simulink model "simulink_both_machines_modified_moore"  (R2019b)
settings: Solver=VariableStepAuto  StartTime=0.0  StopTime=inf  RelTol=1e-3
settings Model: EnablePacing=on  PacingRate=0.250000  Creator=Bishoy Zaky  LastModifiedBy=Bishoy Zaky

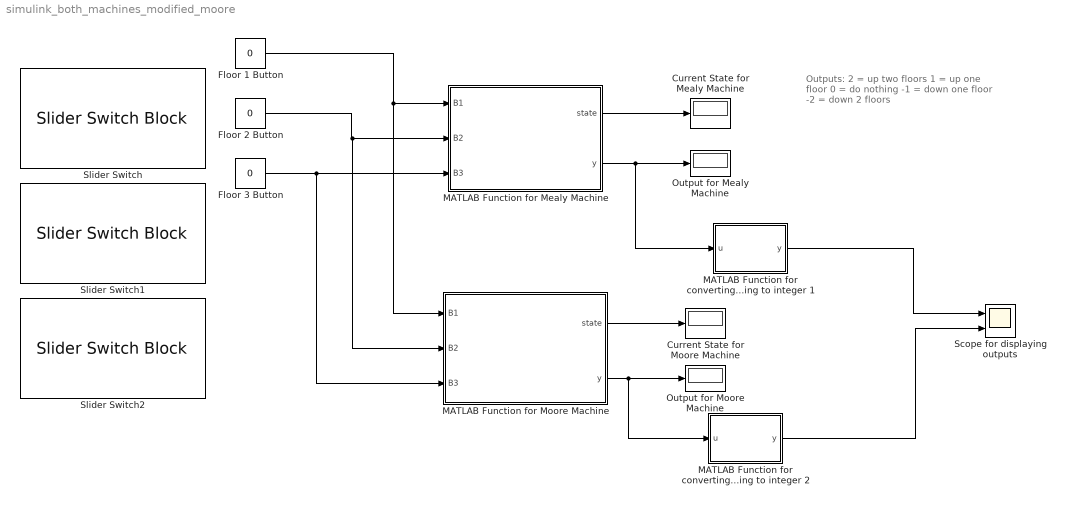
== system simulink_both_machines_modified_moore ==
  note: Outputs:
      | 2 = up two floors
      | 1 = up one floor
      | 0 = do nothing
      | -1 = down one floor
      | -2 = down 2 floors
  Current State for Mealy Machine : Display
  Current State for Moore Machine : Display
  Floor 1 Button : Constant  Value=0
  Floor 2 Button : Constant  Value=0
  Floor 3 Button : Constant  Value=0
  MATLAB Function for Mealy Machine : MATLAB Function  TreatAsAtomicUnit=on
  MATLAB Function for Moore Machine : MATLAB Function  TreatAsAtomicUnit=on
  MATLAB Function for converting output string to integer 1 : MATLAB Function  TreatAsAtomicUnit=on
  MATLAB Function for converting output string to integer 2 : MATLAB Function  TreatAsAtomicUnit=on
  Output for Mealy Machine : Display
  Output for Moore Machine : Display
  Scope for displaying outputs : Scope  NumInputPorts=2
  Slider Switch : SliderSwitchBlock
      settings: Values={{'Off', 'On'}, [0 1]}
  Slider Switch1 : SliderSwitchBlock
      settings: Values={{'Off', 'On'}, [0 1]}
  Slider Switch2 : SliderSwitchBlock
      settings: Values={{'Off', 'On'}, [0 1]}
  wires:
  Floor 1 Button/1 -> MATLAB Function for Moore Machine/1(B1), MATLAB Function for Mealy Machine/1(B1)
  MATLAB Function for converting output string to integer 1/1(y) -> Scope for displaying outputs/1
  Floor 2 Button/1 -> MATLAB Function for Moore Machine/2(B2), MATLAB Function for Mealy Machine/2(B2)
  MATLAB Function for Moore Machine/1(state) -> Current State for Moore Machine/1
  MATLAB Function for converting output string to integer 2/1(y) -> Scope for displaying outputs/2
  MATLAB Function for Mealy Machine/1(state) -> Current State for Mealy Machine/1
  Floor 3 Button/1 -> MATLAB Function for Moore Machine/3(B3), MATLAB Function for Mealy Machine/3(B3)
  MATLAB Function for Moore Machine/2(y) -> Output for Moore Machine/1, MATLAB Function for converting output string to integer 2/1(u)
  MATLAB Function for Mealy Machine/2(y) -> Output for Mealy Machine/1, MATLAB Function for converting output string to integer 1/1(u)

== matlab function simulink_both_machines_modified_moore/MATLAB Function for Moore Machine ==
  data: state output; B1 input; y output; B2 input; B3 input
function [state,y] = fcn(B1,B2,B3)
persistent current_state %state variable that persistes with every function call
if(isempty(current_state)) %initializing the state variable during first function call
    current_state = 1;
end
switch current_state 
    case 1 %state q1 represents being in the first floor
        if(B1) %B1, the first floor button, is pressed
            current_state = 1;
        elseif(B2) %B2, the second floor button, is pressed
            current_state = 4;
        elseif(B3) %B3, the third floor button, is pressed
            current_state = 6;
        end
    case 2 %state q2 represents being in the second floor
        if(B1)
            current_state = 5;
        elseif(B2)
            current_state = 2;
        elseif(B3)
            current_state = 4;
        end
    case 3 %state q3 represents being in the third floor
        if(B1) 
            current_state = 7;
        elseif(B2)
            current_state = 5;
        elseif(B3)
            current_state = 3;
        end
    case 4 %state q4 represents the transition state (first floor to second floor)
        if(B2)
            current_state = 2;
        elseif(B3)
            current_state = 3;
        elseif(B1)
            current_state = 4;
        end
    case 5 %state q5 represents the transition state (second floor to first floor)
        if(B1)
            current_state = 1;
        elseif(B2)
            current_state = 2;
        elseif(B3)
            current_state = 5;
        end
    case 6 %state q6 represents the transition state (first floor to third floor)
        if(B3)
            current_state = 3;
        elseif(B1)
            current_state = 6;    
        elseif(B2)
            current_state = 6;
        end  
    case 7 %state q7 represents the transition state (third floor to first floor)
        if(B1)
            current_state = 1;
        elseif(B2)
            current_state = 7;
        elseif(B3)
            current_state = 7;
        end
end
switch current_state %choose output depending on only the current state
    case 1 
        y = "s"; %elevator remains in place
    case 2
        y = "s";
    case 3
        y = "s";
    case 4
        y = "u1"; %elevator goes up 1 floor
    case 5
        y = "d1";
    case 6
        y = "u2"; %elevator goes up 2 floors
    otherwise
        y = "d2"; %elevator goes down 2 floors
end
state = current_state; %output current state
end

== matlab function simulink_both_machines_modified_moore/MATLAB Function for Mealy Machine ==
  data: state output; B1 input; y output; B2 input; B3 input
function [state,y] = fcn(B1,B2,B3)
persistent current_state %state variable that persistes with every function call
if(isempty(current_state)) %initializing the state variable during first function call
    current_state = 1;
end
switch current_state
    case 1  %state q1 represents being in the first floor
        if(B2) %B2, the second floor button, is pressed
            current_state = 2;
            y = "u1"; %elevator goes up 1 floor
        elseif(B3) %B3, the third floor button, is pressed
            current_state = 3;
            y = "u2"; %elevator goes up 2 floors
        else %B1, the first floor button, is pressed
            current_state = 1;
            y = "s"; %elevator remains in place
        end
    case 2  %state q2 represents being in the second floor
        if(B1)
            current_state = 1;
            y = "d1"; %elevator goes down 1 floor
        elseif(B3)
            current_state = 3;
            y = "u1"; %elevator goes up 1 floor
        else
            current_state = 2;
            y = "s"; %elevator remains in place
        end
    otherwise %otherwise state q3 represents being in the third floor
        if(B1)
            current_state = 1;
            y = "d2"; %elevator goes down 2 floors
        elseif(B2)
            current_state = 2;
            y = "d1"; %elevator goes down 1 floor
        else
            current_state = 3;
            y = "s"; %elevator remains in place
        end
end
state = current_state; %output current state
end

== matlab function simulink_both_machines_modified_moore/MATLAB Function for converting output string to integer 1 ==
  data: u input; y output
function y = fcn(u)
if u == "s"
    y = 0;
elseif u == "u1"
    y = 1;
elseif u == "u2"
    y = 2;
elseif u == "d1"
    y = -1;
else
    y = -2;
end

== matlab function simulink_both_machines_modified_moore/MATLAB Function for converting output string to integer 2 ==
  data: u input; y output
function y = fcn(u)
if u == "s"
    y = 0;
elseif u == "u1"
    y = 1;
elseif u == "u2"
    y = 2;
elseif u == "d1"
    y = -1;
else
    y = -2;
end
